simulink model "untitled"  (R2019a)
settings: Solver=VariableStepAuto  StartTime=0.0  StopTime=10  RelTol=1e-3
values from neighbouring files (symbols this model uses):
  alfa_cu = 3.9 * 10^(-3)    (= 0.0039)    [Datos.m]
  bl = 0    [Datos.m]
  bm = 1.5 * 10^(-5)    (= 1.5e-05)    [Datos.m]
  Cts = 0.818    [Datos.m]
  Id0 = 0.5    [Datos.m]    (also in punto6plot.m)
  Jl = 0.2520    (= 0.252)    [Datos.m]
  Jm = 3.1 * 10^(-6)    (= 3.1e-06)    [Datos.m]
  Kid = 0    [Datos.m]
  Kiq = 0    [Datos.m]
  lambda_m_r = 0.01546    [Datos.m]
  Ld = 6.6e-3    (= 0.0066)    [Datos.m]
  Lls = 0.8e-3    (= 0.0008)    [Datos.m]
  Lq = 5.8e-3    (= 0.0058)    [Datos.m]
  Pp = 3    [Datos.m]
  r = 314.3008    [Datos.m]
  Rts_amb = 146.7    [Datos.m]
  Tlmax = 6.28    [Calculo.m]    (also in Datos.m)
  tstep1 = 0.1    [Calculo.m]    (also in Datos.m)
  tstep2 = 0.3    [Calculo.m]    (also in Datos.m)
  tstep4 = 0.7    [Calculo.m]    (also in Datos.m)
  tstep5 = 0.9    [Calculo.m]    (also in Datos.m)
  Vqsnom = 19.596    [Calculo.m]    (also in Datos.m)
undefined symbols (not defined in the file or in its folder): magnitude
settings Model: Creator=renzo  LastModifiedBy=renzo

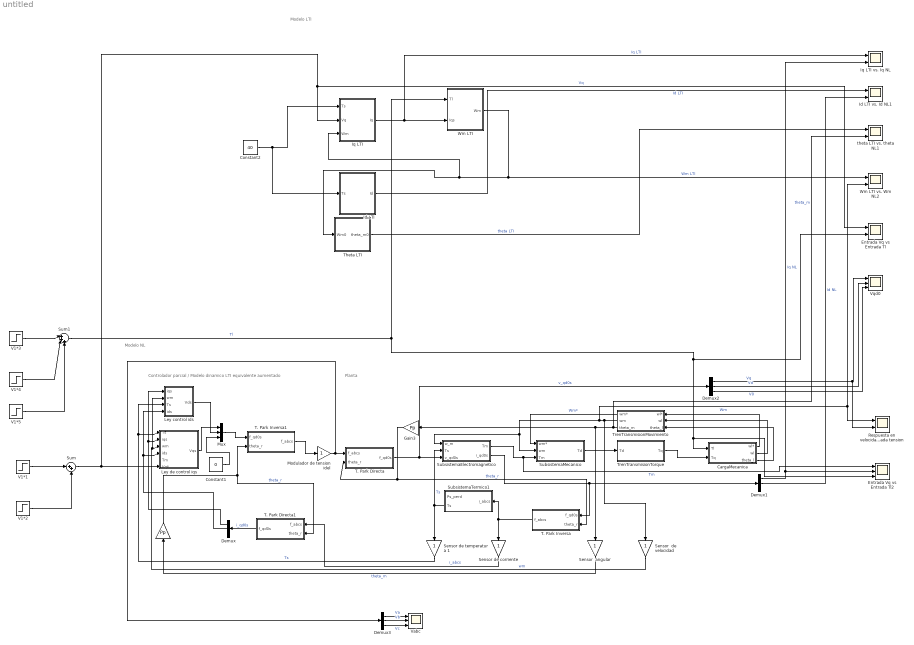
== system untitled ==
  note: Modelo LTI
  note: Modelo NL
  note: Controlador parcial / Modelo dinamico LTI equivalente aumentado
  note: Planta
  " " : Gain  Gain=Pp
  CargaMecanica : Subsystem
  Constant1 : Constant  Value=0
  Constant2 : Constant  Value=40
  Demux{,1..3} (4 alike) : Demux  Outputs=3
  Entrada Vq vs Entrada Tl : Scope  NumInputPorts=2
  Entrada Vq vs Entrada Tl2 : Scope  NumInputPorts=3
  Gain3 : Gain  Gain=Pp
  Id LTI : Subsystem
  Id LTI vs. Id NL1 : Scope  NumInputPorts=2
  Iq LTI : Subsystem
  Iq LTI vs. Iq NL : Scope  NumInputPorts=2
  Ley control ids : Subsystem
  Ley de control iqs : Subsystem
  "Modulador de tension idel " : Gain
  Mux : Mux  Inputs=3
  Respuesta en velocidad vs entrada tension : Scope  NumInputPorts=2
  Sensor  angular : Gain
  Sensor  de velocidad : Gain
  "Sensor de corriente " : Gain
  Sensor de temperatura 1 : Gain
  SubsistemaElectromagnetico : Subsystem
  SubsistemaMecanico : Subsystem
  SubsistemaTermico1 : Subsystem
  Sum : Sum  Inputs=|++
  Sum1 : Sum  Inputs=|+++
  T. Park Directa : Subsystem
  T. Park Directa1 : Subsystem
  T. Park Inversa : Subsystem
  T. Park Inversa1 : Subsystem
  Theta LTI : Subsystem
  TrenTransmisionMovimiento : Subsystem
  TrenTransmisionTorque : Subsystem
  V1*1 : Step  Time=tstep1  After=Vqsnom  SampleTime=0
  V1*2 : Step  Time=tstep4  After=-Vqsnom  SampleTime=0
  V1*3 : Step  Time=tstep2  After=Tlmax  SampleTime=0
  V1*4 : Step  Time=tstep4  After=-2*Tlmax  SampleTime=0
  V1*5 : Step  Time=tstep5  After=Tlmax  SampleTime=0
  Vabc : Scope  NumInputPorts=3
  "Vqd0 " : Scope  NumInputPorts=3
  Wm LTI : Subsystem
  Wm LTI vs. Wm NL2 : Scope  NumInputPorts=2
  theta LTI vs. theta NL1 : Scope  NumInputPorts=2
  wires:
  Wm LTI/1(Wm) -> Theta LTI/1(Wm0), Iq LTI/3(Wm), Wm LTI vs. Wm NL2/1  "Wm LTI"
  Iq LTI/1(Iq) -> Wm LTI/2(Iqs), Iq LTI vs. Iq NL/1  "Iq LTI"
  Theta LTI/1("theta_m0 ") -> theta LTI vs. theta NL1/1  "theta LTI"
  " "/1 -> T. Park Inversa1/2(theta_r), T. Park Directa1/2(theta_r)  "theta_r"
  Constant1/1 -> Mux/3
  TrenTransmisionMovimiento/1(wm*) -> SubsistemaMecanico/1(wm*)  "Wm*"
  T. Park Directa1/1(f_qd0s) -> Demux/1  "i_qd0s"
  Demux1/2 -> Id LTI vs. Id NL1/2  "Id NL"
  Demux1/1 -> Entrada Vq vs Entrada Tl2/2, Iq LTI vs. Iq NL/2  "Iq NL"
  Sensor  angular/1 -> " "/1  "theta_m"
  Gain3/1 -> T. Park Directa/2(theta_r), T. Park Inversa/2(theta_r)  "theta_r"
  T. Park Inversa/1(f_abcs) -> "Sensor de corriente "/1, SubsistemaTermico1/1(i_abcs)
  Ley control ids/1(Vds) -> Mux/2
  TrenTransmisionTorque/1(Tq) -> CargaMecanica/2(Tq)
  Sensor  de velocidad/1 -> Ley control ids/2(wm), Ley de control iqs/3(wm)  "wm"
  T. Park Directa/1(f_qd0s) -> Demux2/1, SubsistemaElectromagnetico/3("v_qd0s ")  "v_qd0s"
  TrenTransmisionMovimiento/3(theta_m) -> theta LTI vs. theta NL1/2, Sensor  angular/1, Gain3/1  "theta_m"
  SubsistemaMecanico/1(Td) -> TrenTransmisionTorque/1(Td)
  "Sensor de corriente "/1 -> T. Park Directa1/1(f_abcs)  "i_abcs"
  Ley de control iqs/1(Vqs) -> Mux/1
  Demux/2 -> Ley control ids/4(ids), Ley de control iqs/4(ids)
  SubsistemaElectromagnetico/2(i_qd0s) -> Demux1/1, T. Park Inversa/1(f_qd0s)
  SubsistemaTermico1/2(Ts) -> SubsistemaElectromagnetico/2(Ts), Sensor de temperatura 1/1  "Ts"
  T. Park Inversa1/1(f_abcs) -> "Modulador de tension idel "/1
  "Modulador de tension idel "/1 -> Demux3/1, T. Park Directa/1(f_abcs)
  Sensor de temperatura 1/1 -> Ley control ids/3(Ts), Ley de control iqs/1(Ts)  "Ts"
  CargaMecanica/1(wl*) -> TrenTransmisionMovimiento/1(wl*)
  Demux/1 -> Ley control ids/1(iqs), Ley de control iqs/2(iqs)
  CargaMecanica/2(wl) -> TrenTransmisionMovimiento/2(wl)
  TrenTransmisionMovimiento/2(wm) -> Sensor  de velocidad/1, Wm LTI vs. Wm NL2/2, Respuesta en velocidad vs entrada tension/1, SubsistemaElectromagnetico/1(w_m), SubsistemaMecanico/2(wm)  "Wm"
  Mux/1 -> T. Park Inversa1/1(f_qd0s)
  CargaMecanica/3(theta_l) -> TrenTransmisionMovimiento/3(theta_l)
  SubsistemaElectromagnetico/1(Tm) -> Entrada Vq vs Entrada Tl2/1, SubsistemaMecanico/3(Tm)  "Tm"
  Demux2/2 -> "Vqd0 "/2  "Vd"
  V1*1/1 -> Sum/1
  V1*2/1 -> Sum/2
  Sum/1 -> Entrada Vq vs Entrada Tl/1, Iq LTI/2("Vq "), Ley de control iqs/6(Vq*)  "Vq"
  V1*3/1 -> Sum1/1
  V1*4/1 -> Sum1/2
  V1*5/1 -> Sum1/3
  Sum1/1 -> Wm LTI/1(Tl), Entrada Vq vs Entrada Tl2/3, CargaMecanica/1(Tl), Entrada Vq vs Entrada Tl/2  "Tl"
  Id LTI/1(Id) -> Id LTI vs. Id NL1/1  "Id LTI"
  Demux2/1 -> Respuesta en velocidad vs entrada tension/2, "Vqd0 "/1  "Vq"
  Demux2/3 -> "Vqd0 "/3  "V0"
  Demux3/1 -> Vabc/1  "Va"
  Demux3/2 -> Vabc/2  "Vb"
  Demux3/3 -> Vabc/3  "Vc"
  Constant2/1 -> Id LTI/1(Ts), Iq LTI/1(Ts)

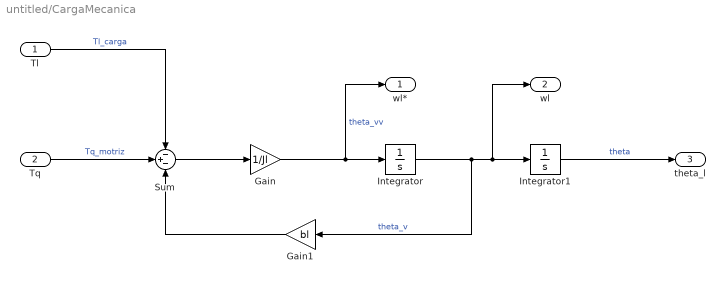
== system untitled/CargaMecanica ==
  Tl : Inport
  Tq : Inport  Port=2
  Gain : Gain  Gain=1/Jl
  Gain1 : Gain  Gain=bl
  Integrator : Integrator
  Integrator1 : Integrator
  Sum : Sum  Inputs=-+-
  wl* : Outport  VectorParamsAs1DForOutWhenUnconnected=on
  wl : Outport  Port=2  VectorParamsAs1DForOutWhenUnconnected=on
  theta_l : Outport  Port=3  VectorParamsAs1DForOutWhenUnconnected=on
  wires:
  Tq/1 -> Sum/2  "Tq_motriz"
  Sum/1 -> Gain/1
  Gain1/1 -> Sum/3
  Tl/1 -> Sum/1  "Tl_carga"
  Integrator/1 -> Gain1/1, wl/1, Integrator1/1  "theta_v"
  Integrator1/1 -> theta_l/1  "theta"
  Gain/1 -> wl*/1, Integrator/1  "theta_vv"

== system untitled/Id LTI ==
  Ts : Inport
  Gain : Gain  Gain=-1/Ld
  Integrator : Integrator  InitialCondition=Id0
  Product : Product
  Rs(t) : Subsystem
  Id : Outport
  wires:
  Rs(t)/1(Rs) -> Product/2
  Ts/1 -> Rs(t)/1(Ts)
  Integrator/1 -> Product/1, Id/1
  Gain/1 -> Integrator/1
  Product/1 -> Gain/1

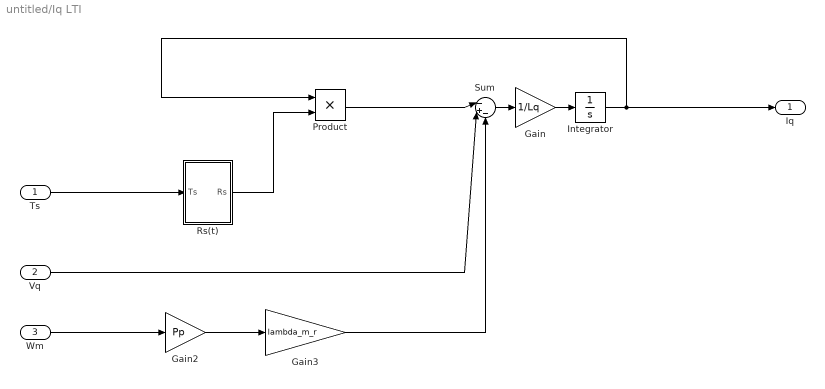
== system untitled/Iq LTI ==
  Ts : Inport
  "Vq " : Inport  Port=2
  Wm : Inport  Port=3
  Gain : Gain  Gain=1/Lq
  Gain2 : Gain  Gain=Pp
  Gain3 : Gain  Gain=lambda_m_r
  Integrator : Integrator
  Product : Product
  Rs(t) : Subsystem
  Sum : Sum  Inputs=|-+-
  Iq : Outport
  wires:
  Rs(t)/1(Rs) -> Product/2
  Ts/1 -> Rs(t)/1(Ts)
  Integrator/1 -> Product/1, Iq/1
  Product/1 -> Sum/1
  Sum/1 -> Gain/1
  "Vq "/1 -> Sum/2
  Wm/1 -> Gain2/1
  Gain2/1 -> Gain3/1
  Gain3/1 -> Sum/3
  Gain/1 -> Integrator/1

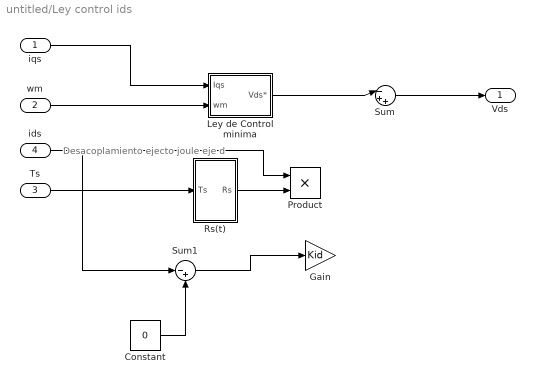
== system untitled/Ley control ids ==
  note: Desacoplamiento ejecto joule eje d
  iqs : Inport
  wm : Inport  Port=2
  Ts : Inport  Port=3
  ids : Inport  Port=4
  Constant : Constant  Value=0
  Gain : Gain  Gain=Kid
  Ley de Control minima : Subsystem
  Product : Product
  Rs(t) : Subsystem
  Sum : Sum  Inputs=|-++
  Sum1 : Sum  Inputs=|-+
  Vds : Outport
  wires:
  wm/1 -> Ley de Control minima/2(wm)
  iqs/1 -> Ley de Control minima/1(Iqs)
  Ley de Control minima/1(Vds*) -> Sum/1
  Rs(t)/1(Rs) -> Product/2
  Sum/1 -> Vds/1
  Ts/1 -> Rs(t)/1(Ts)
  ids/1 -> Sum1/1, Product/1
  Constant/1 -> Sum1/2
  Sum1/1 -> Gain/1

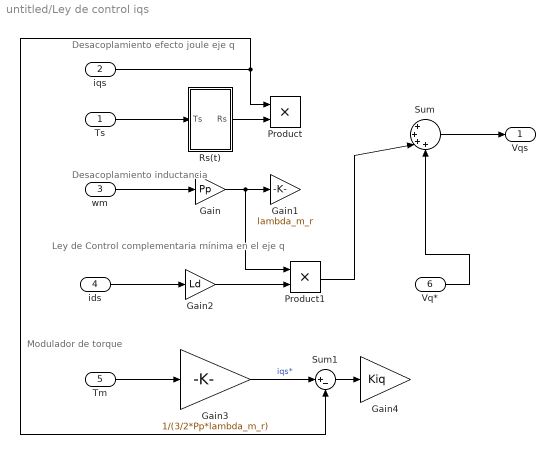
== system untitled/Ley de control iqs ==
  note: Desacoplamiento inductancia
  note: Desacoplamiento efecto joule eje q
  note: Modulador de torque
  note: Ley de Control complementaria mínima en el eje q
  Ts : Inport
  iqs : Inport  Port=2
  wm : Inport  Port=3
  ids : Inport  Port=4
  "Tm " : Inport  Port=5
  Vq* : Inport  Port=6
  Gain : Gain  Gain=Pp
  Gain1 : Gain  Gain=lambda_m_r
  Gain2 : Gain  Gain=Ld
  Gain3 : Gain  Gain=1/(3/2*Pp*lambda_m_r)
  Gain4 : Gain  Gain=Kiq
  Product : Product
  Product1 : Product
  Rs(t) : Subsystem
  Sum : Sum  Inputs=|++++
  Sum1 : Sum  Inputs=|+-
  Vqs : Outport
  wires:
  Rs(t)/1(Rs) -> Product/2
  Ts/1 -> Rs(t)/1(Ts)
  iqs/1 -> Sum1/2, Product/1
  wm/1 -> Gain/1
  Gain/1 -> Product1/1, Gain1/1
  ids/1 -> Gain2/1
  Gain2/1 -> Product1/2
  Product1/1 -> Sum/3
  Sum/1 -> Vqs/1
  "Tm "/1 -> Gain3/1
  Gain3/1 -> Sum1/1  "iqs*"
  Sum1/1 -> Gain4/1
  Vq*/1 -> Sum/4

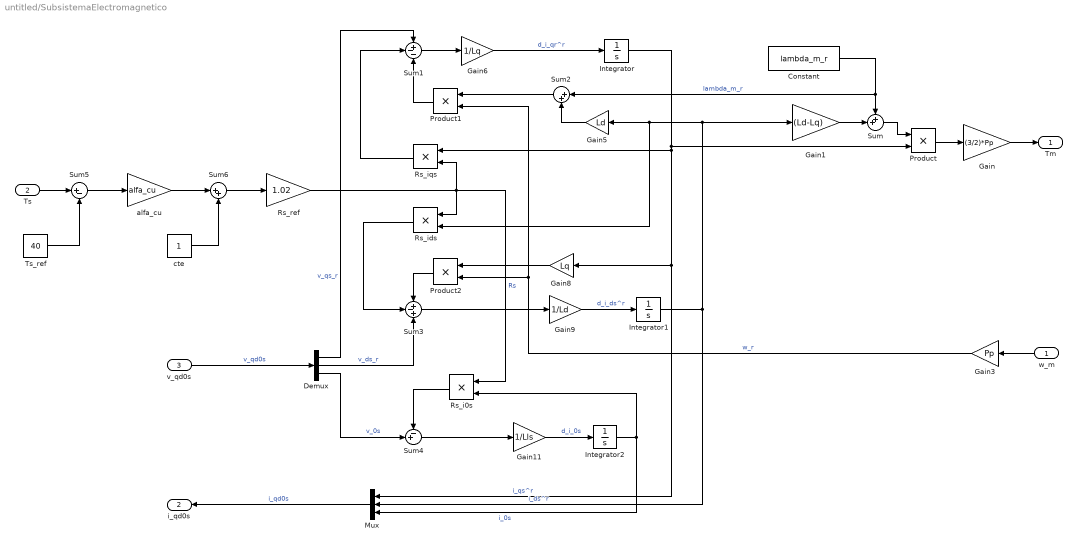
== system untitled/SubsistemaElectromagnetico ==
  w_m : Inport
  Ts : Inport  Port=2
  "v_qd0s " : Inport  Port=3
  Constant : Constant  Value=lambda_m_r
  Demux : Demux  Outputs=3
  Gain : Gain  Gain=(3/2)*Pp
  Gain1 : Gain  Gain=(Ld-Lq)
  Gain11 : Gain  Gain=1/Lls
  Gain3 : Gain  Gain=Pp
  Gain5 : Gain  Gain=Ld
  Gain6 : Gain  Gain=1/Lq
  Gain8 : Gain  Gain=Lq
  Gain9 : Gain  Gain=1/Ld
  Integrator : Integrator
  Integrator1 : Integrator  InitialCondition=Id0
  Integrator2 : Integrator
  Mux : Mux  Inputs=3
  Product : Product
  Product1 : Product
  Product2 : Product
  Rs_i0s : Product
  Rs_ids : Product
  Rs_iqs : Product
  Rs_ref : Gain  Gain=1.02
  Sum : Sum  Inputs=++|
  Sum1 : Sum  Inputs=+--
  Sum2 : Sum  Inputs=|++
  Sum3 : Sum  Inputs=+-+
  Sum4 : Sum  Inputs=-+|
  Sum5 : Sum  Inputs=|+-
  Sum6 : Sum  Inputs=|++
  Ts_ref : Constant  Value=40
  alfa_cu : Gain  Gain=alfa_cu
  cte : Constant
  Tm : Outport  VectorParamsAs1DForOutWhenUnconnected=on
  i_qd0s : Outport  Port=2  VectorParamsAs1DForOutWhenUnconnected=on
  wires:
  Gain/1 -> Tm/1
  Product/1 -> Gain/1
  Integrator/1 -> Product/2, Mux/1, Gain8/1, Rs_iqs/1  "i_qs^r"
  Gain1/1 -> Sum/2
  Integrator1/1 -> Gain5/1, Rs_ids/2, Gain1/1, Mux/2  "i_ds^r"
  Constant/1 -> Sum/1, Sum2/1  "lambda_m_r"
  w_m/1 -> Gain3/1
  "v_qd0s "/1 -> Demux/1  "v_qd0s"
  Demux/1 -> Sum1/1  "v_qs_r"
  Demux/2 -> Sum3/3  "v_ds_r"
  Demux/3 -> Sum4/2  "v_0s"
  Rs_iqs/1 -> Sum1/2
  Product1/1 -> Sum1/3
  Gain3/1 -> Product1/2, Product2/2  "w_r"
  Sum2/1 -> Product1/1
  Gain5/1 -> Sum2/2
  Sum1/1 -> Gain6/1
  Gain6/1 -> Integrator/1  "d_i_qr^r"
  Rs_ids/1 -> Sum3/2
  Product2/1 -> Sum3/1
  Gain8/1 -> Product2/1
  Sum3/1 -> Gain9/1
  Gain9/1 -> Integrator1/1  "d_i_ds^r"
  Rs_i0s/1 -> Sum4/1
  Integrator2/1 -> Rs_i0s/2, Mux/3  "i_0s"
  Sum4/1 -> Gain11/1
  Gain11/1 -> Integrator2/1  "d_i_0s"
  Mux/1 -> i_qd0s/1  "i_qd0s"
  Ts/1 -> Sum5/1
  Ts_ref/1 -> Sum5/2
  Sum5/1 -> alfa_cu/1
  alfa_cu/1 -> Sum6/1
  cte/1 -> Sum6/2
  Sum6/1 -> Rs_ref/1
  Rs_ref/1 -> Rs_ids/1, Rs_i0s/1, Rs_iqs/2  "Rs"
  Sum/1 -> Product/1

== system untitled/SubsistemaMecanico ==
  wm* : Inport
  wm : Inport  Port=2
  Tm : Inport  Port=3
  Gain1 : Gain  Gain=bm
  Gain2 : Gain  Gain=Jm
  Sum : Sum  Inputs=--+
  Td : Outport  VectorParamsAs1DForOutWhenUnconnected=on
  wires:
  wm*/1 -> Gain2/1
  wm/1 -> Gain1/1
  Gain2/1 -> Sum/1
  Gain1/1 -> Sum/2
  Sum/1 -> Td/1
  Tm/1 -> Sum/3

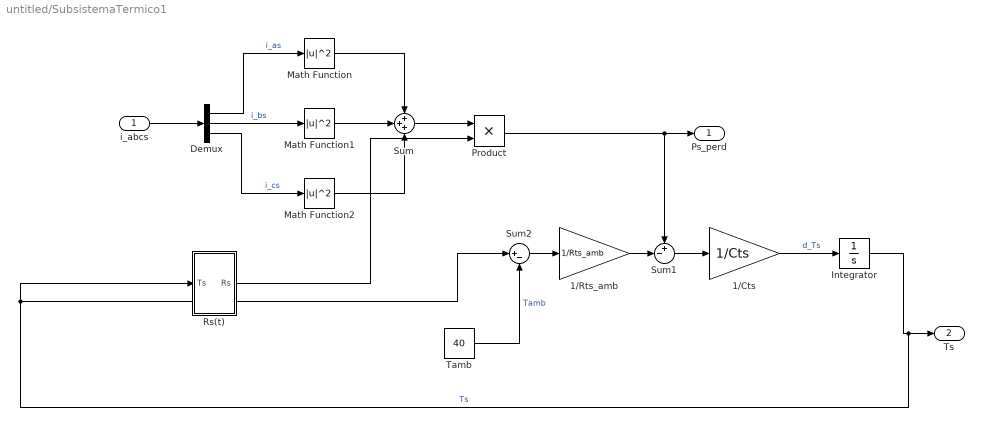
== system untitled/SubsistemaTermico1 ==
  i_abcs : Inport
  1/Cts : Gain  Gain=1/Cts
  1/Rts_amb : Gain  Gain=1/Rts_amb
  Demux : Demux  Outputs=3
  Integrator : Integrator
  Math Function : Math  Operator=magnitude^2  SaturateOnIntegerOverflow=on
  Math Function1 : Math  Operator=magnitude^2  SaturateOnIntegerOverflow=on
  Math Function2 : Math  Operator=magnitude^2  SaturateOnIntegerOverflow=on
  Product : Product
  Rs(t) : Subsystem
  Sum : Sum  Inputs=3
  Sum1 : Sum  Inputs=+-|
  Sum2 : Sum  Inputs=|+-
  Tamb : Constant  Value=40
  Ps_perd : Outport  VectorParamsAs1DForOutWhenUnconnected=on
  Ts : Outport  Port=2  VectorParamsAs1DForOutWhenUnconnected=on
  wires:
  i_abcs/1 -> Demux/1
  Demux/1 -> Math Function/1  "i_as"
  Demux/2 -> Math Function1/1  "i_bs"
  Demux/3 -> Math Function2/1  "i_cs"
  Math Function1/1 -> Sum/2
  Math Function/1 -> Sum/1
  Math Function2/1 -> Sum/3
  Sum/1 -> Product/1
  Product/1 -> Sum1/1, Ps_perd/1
  Tamb/1 -> Sum2/2  "Tamb"
  Sum2/1 -> 1/Rts_amb/1
  1/Rts_amb/1 -> Sum1/2
  Sum1/1 -> 1/Cts/1
  1/Cts/1 -> Integrator/1  "d_Ts"
  Integrator/1 -> Rs(t)/1(Ts), Sum2/1, Ts/1  "Ts"
  Rs(t)/1(Rs) -> Product/2

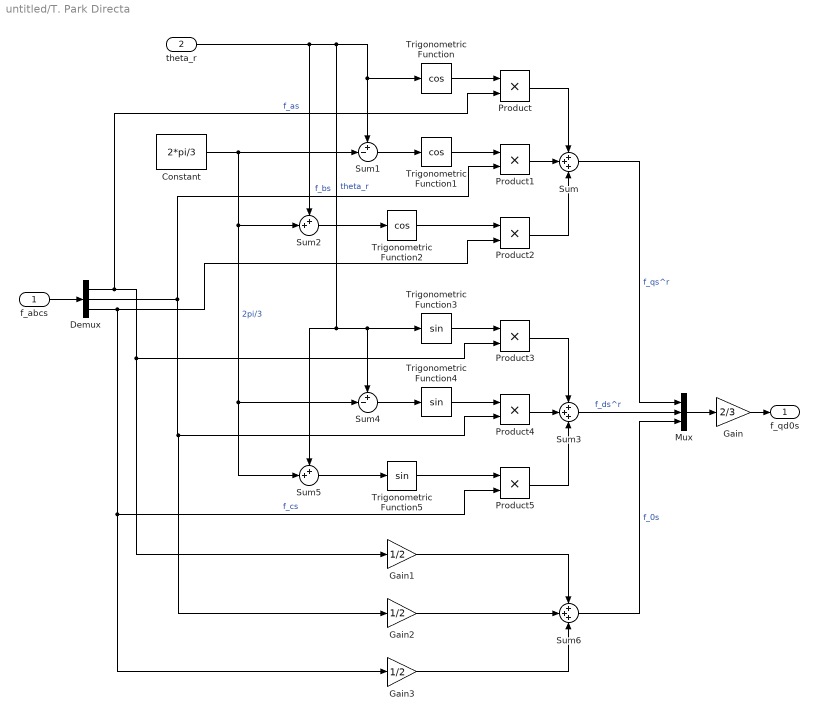
== system untitled/T. Park Directa ==
  f_abcs : Inport
  theta_r : Inport  Port=2
  Constant : Constant  Value=2*pi/3
  Demux : Demux  Outputs=3
  Gain : Gain  Gain=2/3
  Gain1 : Gain  Gain=1/2
  Gain2 : Gain  Gain=1/2
  Gain3 : Gain  Gain=1/2
  Mux : Mux  Inputs=3
  Product{,1..5} (6 alike) : Product
  Sum : Sum  Inputs=3
  Sum1 : Sum  Inputs=+-|
  Sum2 : Sum  Inputs=++|
  Sum3 : Sum  Inputs=3
  Sum4 : Sum  Inputs=+-|
  Sum5 : Sum  Inputs=++|
  Sum6 : Sum  Inputs=3
  Trigonometric Function : Trigonometry  Operator=cos
  Trigonometric Function1 : Trigonometry  Operator=cos
  Trigonometric Function2 : Trigonometry  Operator=cos
  Trigonometric Function3 : Trigonometry
  Trigonometric Function4 : Trigonometry
  Trigonometric Function5 : Trigonometry
  f_qd0s : Outport  VectorParamsAs1DForOutWhenUnconnected=on
  wires:
  Mux/1 -> Gain/1
  f_abcs/1 -> Demux/1
  Demux/1 -> Gain1/1, Product3/2, Product/2  "f_as"
  Demux/2 -> Gain2/1, Product4/2, Product1/2  "f_bs"
  Demux/3 -> Gain3/1, Product5/2, Product2/2  "f_cs"
  Sum/1 -> Mux/1  "f_qs^r"
  Gain/1 -> f_qd0s/1
  Trigonometric Function/1 -> Product/1
  Product/1 -> Sum/1
  Sum1/1 -> Trigonometric Function1/1
  Constant/1 -> Sum5/2, Sum4/2, Sum2/2, Sum1/2  "2pi/3"
  Trigonometric Function1/1 -> Product1/1
  Product1/1 -> Sum/2
  Product2/1 -> Sum/3
  Trigonometric Function2/1 -> Product2/1
  Sum2/1 -> Trigonometric Function2/1
  Product4/1 -> Sum3/2
  Trigonometric Function5/1 -> Product5/1
  Sum5/1 -> Trigonometric Function5/1
  Product5/1 -> Sum3/3
  Product3/1 -> Sum3/1
  Trigonometric Function4/1 -> Product4/1
  Sum4/1 -> Trigonometric Function4/1
  Sum3/1 -> Mux/2  "f_ds^r"
  Trigonometric Function3/1 -> Product3/1
  theta_r/1 -> Sum5/1, Sum4/1, Trigonometric Function3/1, Trigonometric Function/1, Sum1/1, Sum2/1  "theta_r"
  Sum6/1 -> Mux/3  "f_0s"
  Gain3/1 -> Sum6/3
  Gain1/1 -> Sum6/1
  Gain2/1 -> Sum6/2

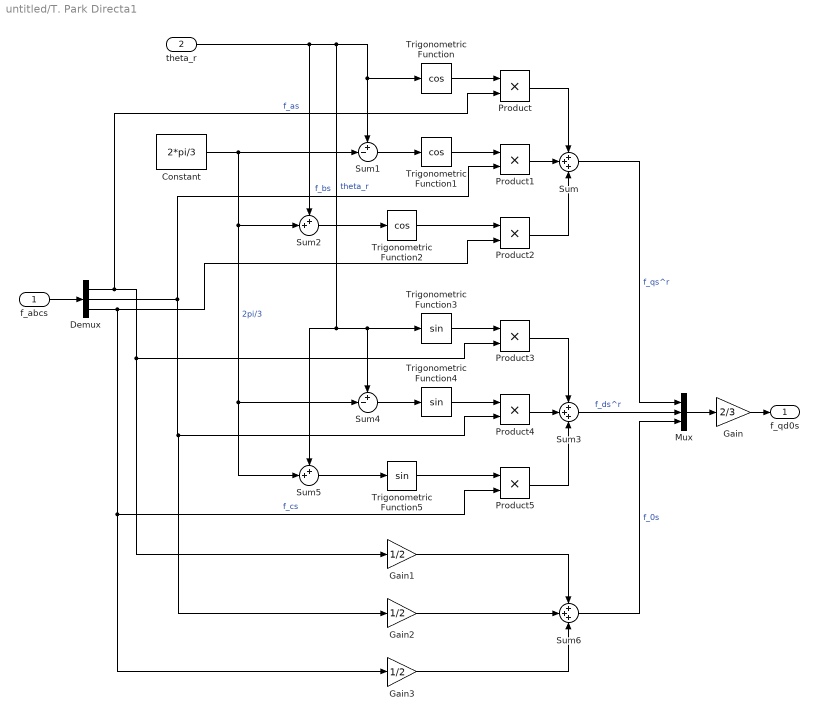
== system untitled/T. Park Directa1 ==
  f_abcs : Inport
  theta_r : Inport  Port=2
  Constant : Constant  Value=2*pi/3
  Demux : Demux  Outputs=3
  Gain : Gain  Gain=2/3
  Gain1 : Gain  Gain=1/2
  Gain2 : Gain  Gain=1/2
  Gain3 : Gain  Gain=1/2
  Mux : Mux  Inputs=3
  Product{,1..5} (6 alike) : Product
  Sum : Sum  Inputs=3
  Sum1 : Sum  Inputs=+-|
  Sum2 : Sum  Inputs=++|
  Sum3 : Sum  Inputs=3
  Sum4 : Sum  Inputs=+-|
  Sum5 : Sum  Inputs=++|
  Sum6 : Sum  Inputs=3
  Trigonometric Function : Trigonometry  Operator=cos
  Trigonometric Function1 : Trigonometry  Operator=cos
  Trigonometric Function2 : Trigonometry  Operator=cos
  Trigonometric Function3 : Trigonometry
  Trigonometric Function4 : Trigonometry
  Trigonometric Function5 : Trigonometry
  f_qd0s : Outport  VectorParamsAs1DForOutWhenUnconnected=on
  wires:
  Mux/1 -> Gain/1
  f_abcs/1 -> Demux/1
  Demux/1 -> Gain1/1, Product3/2, Product/2  "f_as"
  Demux/2 -> Gain2/1, Product4/2, Product1/2  "f_bs"
  Demux/3 -> Gain3/1, Product5/2, Product2/2  "f_cs"
  Sum/1 -> Mux/1  "f_qs^r"
  Gain/1 -> f_qd0s/1
  Trigonometric Function/1 -> Product/1
  Product/1 -> Sum/1
  Sum1/1 -> Trigonometric Function1/1
  Constant/1 -> Sum5/2, Sum4/2, Sum2/2, Sum1/2  "2pi/3"
  Trigonometric Function1/1 -> Product1/1
  Product1/1 -> Sum/2
  Product2/1 -> Sum/3
  Trigonometric Function2/1 -> Product2/1
  Sum2/1 -> Trigonometric Function2/1
  Product4/1 -> Sum3/2
  Trigonometric Function5/1 -> Product5/1
  Sum5/1 -> Trigonometric Function5/1
  Product5/1 -> Sum3/3
  Product3/1 -> Sum3/1
  Trigonometric Function4/1 -> Product4/1
  Sum4/1 -> Trigonometric Function4/1
  Sum3/1 -> Mux/2  "f_ds^r"
  Trigonometric Function3/1 -> Product3/1
  theta_r/1 -> Sum5/1, Sum4/1, Trigonometric Function3/1, Trigonometric Function/1, Sum1/1, Sum2/1  "theta_r"
  Sum6/1 -> Mux/3  "f_0s"
  Gain3/1 -> Sum6/3
  Gain1/1 -> Sum6/1
  Gain2/1 -> Sum6/2

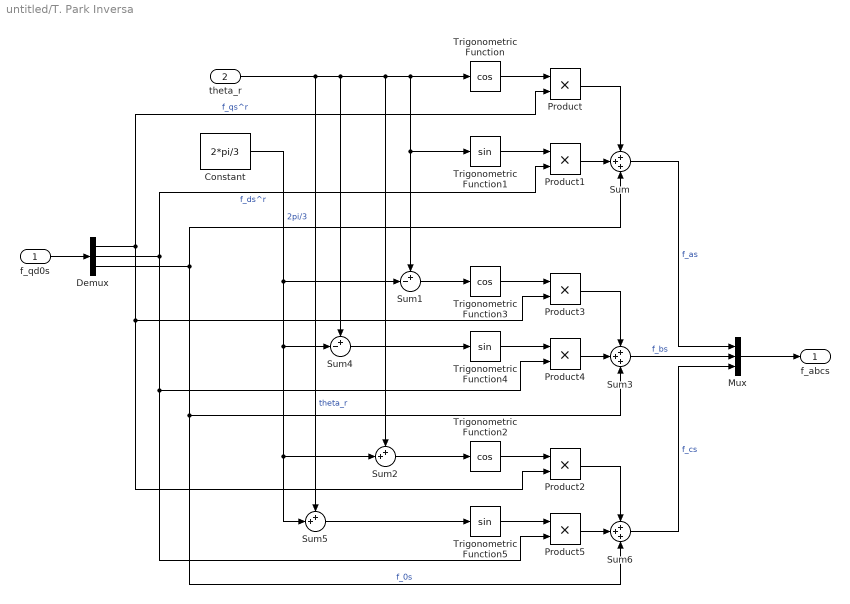
== system untitled/T. Park Inversa ==
  f_qd0s : Inport
  theta_r : Inport  Port=2
  Constant : Constant  Value=2*pi/3
  Demux : Demux  Outputs=3
  Mux : Mux  Inputs=3
  Product{,1..5} (6 alike) : Product
  Sum : Sum  Inputs=3
  Sum1 : Sum  Inputs=+-|
  Sum2 : Sum  Inputs=++|
  Sum3 : Sum  Inputs=3
  Sum4 : Sum  Inputs=+-|
  Sum5 : Sum  Inputs=++|
  Sum6 : Sum  Inputs=3
  Trigonometric Function : Trigonometry  Operator=cos
  Trigonometric Function1 : Trigonometry
  Trigonometric Function2 : Trigonometry  Operator=cos
  Trigonometric Function3 : Trigonometry  Operator=cos
  Trigonometric Function4 : Trigonometry
  Trigonometric Function5 : Trigonometry
  f_abcs : Outport  VectorParamsAs1DForOutWhenUnconnected=on
  wires:
  Trigonometric Function4/1 -> Product4/1
  f_qd0s/1 -> Demux/1
  Trigonometric Function/1 -> Product/1
  Constant/1 -> Sum1/2, Sum4/2, Sum2/2, Sum5/2  "2pi/3"
  Product1/1 -> Sum/2
  Mux/1 -> f_abcs/1
  Sum6/1 -> Mux/3  "f_cs"
  Product/1 -> Sum/1
  theta_r/1 -> Trigonometric Function/1, Trigonometric Function1/1, Sum1/1, Sum2/1, Sum4/1, Sum5/1  "theta_r"
  Product4/1 -> Sum3/2
  Sum3/1 -> Mux/2  "f_bs"
  Trigonometric Function1/1 -> Product1/1
  Sum/1 -> Mux/1  "f_as"
  Trigonometric Function3/1 -> Product3/1
  Product3/1 -> Sum3/1
  Sum4/1 -> Trigonometric Function4/1
  Demux/1 -> Product2/2, Product3/2, Product/2  "f_qs^r"
  Demux/2 -> Product5/2, Product4/2, Product1/2  "f_ds^r"
  Demux/3 -> Sum/3, Sum6/3, Sum3/3  "f_0s"
  Sum1/1 -> Trigonometric Function3/1
  Sum5/1 -> Trigonometric Function5/1
  Trigonometric Function5/1 -> Product5/1
  Trigonometric Function2/1 -> Product2/1
  Product2/1 -> Sum6/1
  Product5/1 -> Sum6/2
  Sum2/1 -> Trigonometric Function2/1

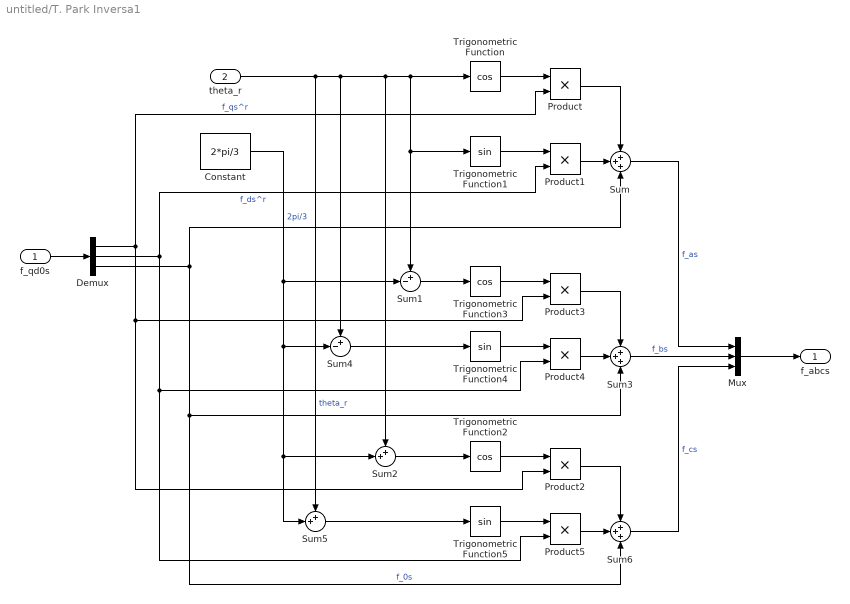
== system untitled/T. Park Inversa1 ==
  f_qd0s : Inport
  theta_r : Inport  Port=2
  Constant : Constant  Value=2*pi/3
  Demux : Demux  Outputs=3
  Mux : Mux  Inputs=3
  Product{,1..5} (6 alike) : Product
  Sum : Sum  Inputs=3
  Sum1 : Sum  Inputs=+-|
  Sum2 : Sum  Inputs=++|
  Sum3 : Sum  Inputs=3
  Sum4 : Sum  Inputs=+-|
  Sum5 : Sum  Inputs=++|
  Sum6 : Sum  Inputs=3
  Trigonometric Function : Trigonometry  Operator=cos
  Trigonometric Function1 : Trigonometry
  Trigonometric Function2 : Trigonometry  Operator=cos
  Trigonometric Function3 : Trigonometry  Operator=cos
  Trigonometric Function4 : Trigonometry
  Trigonometric Function5 : Trigonometry
  f_abcs : Outport  VectorParamsAs1DForOutWhenUnconnected=on
  wires:
  Trigonometric Function4/1 -> Product4/1
  f_qd0s/1 -> Demux/1
  Trigonometric Function/1 -> Product/1
  Constant/1 -> Sum1/2, Sum4/2, Sum2/2, Sum5/2  "2pi/3"
  Product1/1 -> Sum/2
  Mux/1 -> f_abcs/1
  Sum6/1 -> Mux/3  "f_cs"
  Product/1 -> Sum/1
  theta_r/1 -> Trigonometric Function/1, Trigonometric Function1/1, Sum1/1, Sum2/1, Sum4/1, Sum5/1  "theta_r"
  Product4/1 -> Sum3/2
  Sum3/1 -> Mux/2  "f_bs"
  Trigonometric Function1/1 -> Product1/1
  Sum/1 -> Mux/1  "f_as"
  Trigonometric Function3/1 -> Product3/1
  Product3/1 -> Sum3/1
  Sum4/1 -> Trigonometric Function4/1
  Demux/1 -> Product2/2, Product3/2, Product/2  "f_qs^r"
  Demux/2 -> Product5/2, Product4/2, Product1/2  "f_ds^r"
  Demux/3 -> Sum/3, Sum6/3, Sum3/3  "f_0s"
  Sum1/1 -> Trigonometric Function3/1
  Sum5/1 -> Trigonometric Function5/1
  Trigonometric Function5/1 -> Product5/1
  Trigonometric Function2/1 -> Product2/1
  Product2/1 -> Sum6/1
  Product5/1 -> Sum6/2
  Sum2/1 -> Trigonometric Function2/1

== system untitled/Theta LTI ==
  Wm0 : Inport
  Integrator : Integrator
  "theta_m0 " : Outport
  wires:
  Wm0/1 -> Integrator/1
  Integrator/1 -> "theta_m0 "/1

== system untitled/TrenTransmisionMovimiento ==
  wl* : Inport
  wl : Inport  Port=2
  theta_l : Inport  Port=3
  Gain : Gain  Gain=r
  Gain2 : Gain  Gain=r
  Gain3 : Gain  Gain=r
  wm* : Outport  VectorParamsAs1DForOutWhenUnconnected=on
  wm : Outport  Port=2  VectorParamsAs1DForOutWhenUnconnected=on
  theta_m : Outport  Port=3  VectorParamsAs1DForOutWhenUnconnected=on
  wires:
  Gain2/1 -> wm*/1
  wl/1 -> Gain/1
  wl*/1 -> Gain2/1
  Gain/1 -> wm/1
  theta_l/1 -> Gain3/1
  Gain3/1 -> theta_m/1

== system untitled/TrenTransmisionTorque ==
  Td : Inport
  Gain1 : Gain  Gain=r
  Tq : Outport  VectorParamsAs1DForOutWhenUnconnected=on
  wires:
  Td/1 -> Gain1/1
  Gain1/1 -> Tq/1

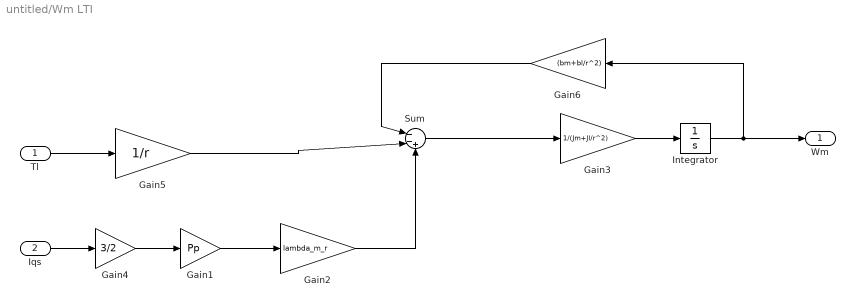
== system untitled/Wm LTI ==
  Tl : Inport
  Iqs : Inport  Port=2
  Gain1 : Gain  Gain=Pp
  Gain2 : Gain  Gain=lambda_m_r
  Gain3 : Gain  Gain=1/(Jm+Jl/r^2)
  Gain4 : Gain  Gain=3/2
  Gain5 : Gain  Gain=1/r
  Gain6 : Gain  Gain=(bm+bl/r^2)
  Integrator : Integrator
  Sum : Sum  Inputs=|--+
  Wm : Outport
  wires:
  Gain1/1 -> Gain2/1
  Integrator/1 -> Gain6/1, Wm/1
  Iqs/1 -> Gain4/1
  Gain4/1 -> Gain1/1
  Gain2/1 -> Sum/3
  Tl/1 -> Gain5/1
  Gain5/1 -> Sum/2
  Sum/1 -> Gain3/1
  Gain3/1 -> Integrator/1
  Gain6/1 -> Sum/1

== system untitled/Id LTI/Rs(t) ==
  Ts : Inport
  Rs_ref : Gain  Gain=1.02
  Sum5 : Sum  Inputs=|+-
  Sum6 : Sum  Inputs=|++
  Ts_ref : Constant  Value=40
  alfa_cu : Gain  Gain=alfa_cu
  cte : Constant
  Rs : Outport
  wires:
  alfa_cu/1 -> Sum6/1
  Sum6/1 -> Rs_ref/1
  Rs_ref/1 -> Rs/1  "Rs"
  Ts_ref/1 -> Sum5/2
  cte/1 -> Sum6/2
  Ts/1 -> Sum5/1
  Sum5/1 -> alfa_cu/1

== system untitled/Iq LTI/Rs(t) ==
  Ts : Inport
  Rs_ref : Gain  Gain=1.02
  Sum5 : Sum  Inputs=|+-
  Sum6 : Sum  Inputs=|++
  Ts_ref : Constant  Value=40
  alfa_cu : Gain  Gain=alfa_cu
  cte : Constant
  Rs : Outport
  wires:
  alfa_cu/1 -> Sum6/1
  Sum6/1 -> Rs_ref/1
  Rs_ref/1 -> Rs/1  "Rs"
  Ts_ref/1 -> Sum5/2
  cte/1 -> Sum6/2
  Ts/1 -> Sum5/1
  Sum5/1 -> alfa_cu/1

== system untitled/Ley control ids/Ley de Control minima ==
  Iqs : Inport
  wm : Inport  Port=2
  " 1" : Gain  Gain=Lq
  " 2" : Gain  Gain=Pp
  Product : Product
  Vds* : Outport
  wires:
  Iqs/1 -> " 1"/1  "iqs"
  " 1"/1 -> " 2"/1
  " 2"/1 -> Product/2
  wm/1 -> Product/1  "iqs"
  Product/1 -> Vds*/1

== system untitled/Ley control ids/Rs(t) ==
  Ts : Inport
  Rs_ref : Gain  Gain=1.02
  Sum5 : Sum  Inputs=|+-
  Sum6 : Sum  Inputs=|++
  Ts_ref : Constant  Value=40
  alfa_cu : Gain  Gain=alfa_cu
  cte : Constant
  Rs : Outport
  wires:
  alfa_cu/1 -> Sum6/1
  Sum6/1 -> Rs_ref/1
  Rs_ref/1 -> Rs/1  "Rs"
  Ts_ref/1 -> Sum5/2
  cte/1 -> Sum6/2
  Ts/1 -> Sum5/1
  Sum5/1 -> alfa_cu/1

== system untitled/Ley de control iqs/Rs(t) ==
  Ts : Inport
  Rs_ref : Gain  Gain=1.02
  Sum5 : Sum  Inputs=|+-
  Sum6 : Sum  Inputs=|++
  Ts_ref : Constant  Value=40
  alfa_cu : Gain  Gain=alfa_cu
  cte : Constant
  Rs : Outport
  wires:
  alfa_cu/1 -> Sum6/1
  Sum6/1 -> Rs_ref/1
  Rs_ref/1 -> Rs/1  "Rs"
  Ts_ref/1 -> Sum5/2
  cte/1 -> Sum6/2
  Ts/1 -> Sum5/1
  Sum5/1 -> alfa_cu/1

== system untitled/SubsistemaTermico1/Rs(t) ==
  Ts : Inport
  Rs_ref : Gain  Gain=1.02
  Sum5 : Sum  Inputs=|+-
  Sum6 : Sum  Inputs=|++
  Ts_ref : Constant  Value=40
  alfa_cu : Gain  Gain=alfa_cu
  cte : Constant
  Rs : Outport
  wires:
  alfa_cu/1 -> Sum6/1
  Sum6/1 -> Rs_ref/1
  Rs_ref/1 -> Rs/1  "Rs"
  Ts_ref/1 -> Sum5/2
  cte/1 -> Sum6/2
  Ts/1 -> Sum5/1
  Sum5/1 -> alfa_cu/1
